simulink model "steeringwheel_clean"  (Simulink 9.2)
settings: Solver=ode45  StartTime=0.0  StopTime=60  MaxStep=1e-3  RelTol=1e-6
settings Model: Creator=jinwooro  LastModifiedBy=jinwooro
settings DataIOCC: LimitDataPoints=off  SaveFormat=Dataset  SignalLoggingSaveFormat=Dataset
settings OptimizationCC: LifeSpan=auto
settings DebuggingCC: UnderspecifiedInitializationDetection=Simplified  MergeDetectMultiDrivingBlocksExec=error  FcnCallInpInsideContextMsg=error  StateNameClashWarn=none  SFUnexpectedBacktrackingDiag=error  SFNoUnconditionalDefaultTransitionDiag=error  SFExecutionAtInitializationDiag=warning
settings HardwareCC: ProdBitPerPointer=64  ProdBitPerSizeT=64  ProdBitPerPtrDiffT=64  ProdLargestAtomicFloat=Float  ProdIntDivRoundTo=Zero  ProdEndianess=LittleEndian  ProdWordSize=64  ProdHWDeviceType=Intel->x86-64 (Windows64)
settings ModelReferenceCC: PropagateSignalLabelsOutOfModel=on
settings SFSimCC: SimUseLocalCustomCode=on
settings RTWCC: RTWUseLocalCustomCode=on
settings CodeAppCC: StateflowObjectComments=off
settings GRTTargetCC: TargetLangStandard=C99 (ISO)  GeneratePreprocessorConditionals=Use local settings  CombineOutputUpdateFcns=on  GRTInterface=off
settings ConfigComp: CovMetricSettings=dwe  CovHtmlReporting=off  CovSaveCumulativeToWorkspaceVar=off  CovSaveSingleToWorkspaceVar=off  CovExternalEMLEnable=on

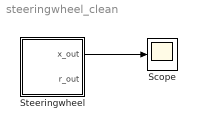
== system steeringwheel_clean ==
  Scope : Scope
  Steeringwheel : Stateflow chart  TreatAsAtomicUnit=on
  wires:
  Steeringwheel/1(x_out) -> Scope/1

== stateflow chart Steeringwheel ==
  settings: updateMethod=CONTINUOUS
  state LeftTurn
    du:
    r_dot = 1;
    r_out = r;
    x_out = cos(r);
  state RightTurn
    du:
    r_dot = -3*pi;
    r_out = r;
    x_out = cos(r);
  (default) -> LeftTurn : {r = 0;}
  LeftTurn -> RightTurn : [cos(r) <= -0.99]
  RightTurn -> LeftTurn : [cos(r) >= 0.99]
  data: r local double; x_out output double; r_out output double
  data r settings: updateMethod=SF_CONTINUOUS_TIME_DATA
